simulink model "ControlSystem"  (R2024a)
settings: Solver=FixedStepAuto  StartTime=0.0  StopTime=data.Timestamp(end)  FixedStep=1/60  RelTol=1e-3
values from neighbouring files (symbols this model uses):
  a_denum = exp(-dt/tau_act)    [SimParam.m]
  a_num = 1 - a_denum    [SimParam.m]
  dt = 1/60    (= 0.0166666666667)    [SimParam.m]
  dx = g.dx    [SimParam.m]
  dy = g.dy    [SimParam.m]
  g_a = p.g    [SimParam.m]
  gx = g.gx    [SimParam.m]
  gy = g.gy    [SimParam.m]
  k_heave = 0.05    [SimParam.m]
  k_surge = 0.15    [SimParam.m]
  k_sway = 0.05    [SimParam.m]
  L_i0 = 0.1    [SimParam.m]
  L_max = 0.1    [SimParam.m]
  L_min = -0.1    [SimParam.m]
  max_deg_Surge = 10    [SimParam.m]
  max_deg_Sway = 5    [SimParam.m]
  thickness = g.t    [SimParam.m]
undefined symbols (not defined in the file or in its folder): DiscIntNeverNeededParam
settings Model: Creator=gusta  LastModifiedBy=gusta

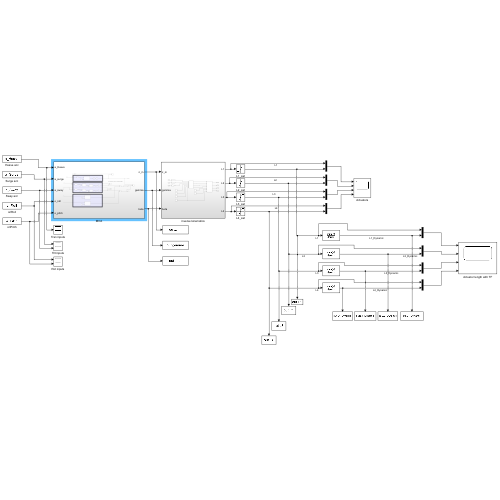
[thumbnail: Simulink's stored preview of the top-level diagram]
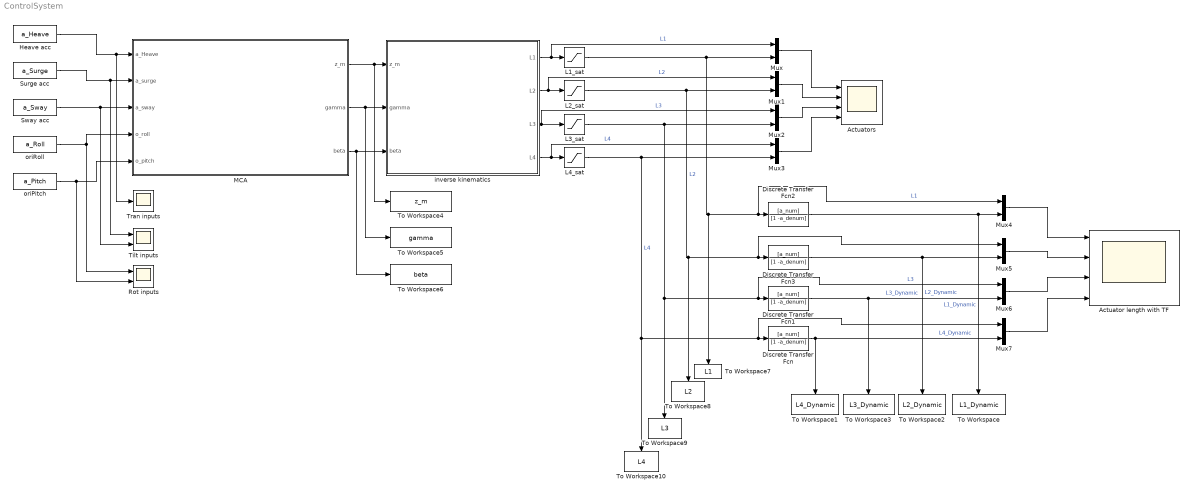
== system ControlSystem ==
  Actuator length with TF : Scope  NumInputPorts=4
  Actuators : Scope  NumInputPorts=4
  Discrete Transfer Fcn{,1..3} (4 alike) : DiscreteTransferFcn  Numerator=[a_num]  Denominator=[1 -a_denum]
  Heave acc : FromWorkspace  VariableName=a_Heave
  L1_sat : Saturate  UpperLimit=L_max  LowerLimit=L_min  ZeroCross=off
  L2_sat : Saturate  UpperLimit=L_max  LowerLimit=L_min  ZeroCross=off
  L3_sat : Saturate  UpperLimit=L_max  LowerLimit=L_min  ZeroCross=off
  L4_sat : Saturate  UpperLimit=L_max  LowerLimit=L_min  ZeroCross=off
  MCA : Subsystem
  Mux{,1..7} (8 alike) : Mux  Inputs=2
  Rot inputs : Scope  NumInputPorts=2
  Surge acc : FromWorkspace  VariableName=a_Surge
  Sway acc : FromWorkspace  VariableName=a_Sway
  Tilt inputs : Scope  NumInputPorts=2
  To Workspace : ToWorkspace  VariableName=L1_Dynamic  SaveFormat=Timeseries  SampleTime=-1
  To Workspace1 : ToWorkspace  VariableName=L4_Dynamic  SaveFormat=Timeseries  SampleTime=-1
  To Workspace10 : ToWorkspace  VariableName=L4  SaveFormat=Timeseries  SampleTime=-1
  To Workspace2 : ToWorkspace  VariableName=L2_Dynamic  SaveFormat=Timeseries  SampleTime=-1
  To Workspace3 : ToWorkspace  VariableName=L3_Dynamic  SaveFormat=Timeseries  SampleTime=-1
  To Workspace4 : ToWorkspace  VariableName=z_m  SaveFormat=Timeseries  SampleTime=-1
  To Workspace5 : ToWorkspace  VariableName=gamma  SaveFormat=Timeseries  SampleTime=-1
  To Workspace6 : ToWorkspace  VariableName=beta  SaveFormat=Timeseries  SampleTime=-1
  To Workspace7 : ToWorkspace  VariableName=L1  SaveFormat=Timeseries  SampleTime=-1
  To Workspace8 : ToWorkspace  VariableName=L2  SaveFormat=Timeseries  SampleTime=-1
  To Workspace9 : ToWorkspace  VariableName=L3  SaveFormat=Timeseries  SampleTime=-1
  Tran inputs : Scope
  inverse kinematics : Subsystem
  oriPitch : FromWorkspace  VariableName=a_Pitch
  oriRoll : FromWorkspace  VariableName=a_Roll
  wires:
  Heave acc/1 -> Tran inputs/1, MCA/1(a_Heave)
  Surge acc/1 -> Tilt inputs/1, MCA/2(a_surge)
  Sway acc/1 -> Tilt inputs/2, MCA/3(a_sway)
  oriRoll/1 -> Rot inputs/1, MCA/4(o_roll)
  oriPitch/1 -> Rot inputs/2, MCA/5(o_pitch)
  MCA/1(z_m) -> To Workspace4/1, inverse kinematics/1(z_m)
  MCA/2(gamma) -> To Workspace5/1, inverse kinematics/2(gamma)
  MCA/3(beta) -> To Workspace6/1, inverse kinematics/3(beta)
  inverse kinematics/4(L4) -> Mux3/1, L4_sat/1  "L4"
  inverse kinematics/3(L3) -> Mux2/1, L3_sat/1  "L3"
  inverse kinematics/2(L2) -> Mux1/1, L2_sat/1  "L2"
  L1_sat/1 -> Mux/2, Mux4/1, Discrete Transfer Fcn2/1, To Workspace7/1  "L1"
  L2_sat/1 -> Mux1/2, Discrete Transfer Fcn3/1, Mux5/1, To Workspace8/1  "L2"
  L3_sat/1 -> Mux2/2, Discrete Transfer Fcn1/1, Mux6/1, To Workspace9/1  "L3"
  L4_sat/1 -> Mux3/2, Mux7/1, Discrete Transfer Fcn/1, To Workspace10/1  "L4"
  inverse kinematics/1(L1) -> Mux/1, L1_sat/1  "L1"
  Mux/1 -> Actuators/1
  Mux1/1 -> Actuators/2
  Mux2/1 -> Actuators/3
  Mux3/1 -> Actuators/4
  Discrete Transfer Fcn2/1 -> To Workspace/1, Mux4/2  "L1_Dynamic"
  Discrete Transfer Fcn3/1 -> Mux5/2, To Workspace2/1  "L2_Dynamic"
  Discrete Transfer Fcn1/1 -> Mux6/2, To Workspace3/1  "L3_Dynamic"
  Discrete Transfer Fcn/1 -> Mux7/2, To Workspace1/1  "L4_Dynamic"
  Mux4/1 -> Actuator length with TF/1
  Mux5/1 -> Actuator length with TF/2
  Mux6/1 -> Actuator length with TF/3
  Mux7/1 -> Actuator length with TF/4

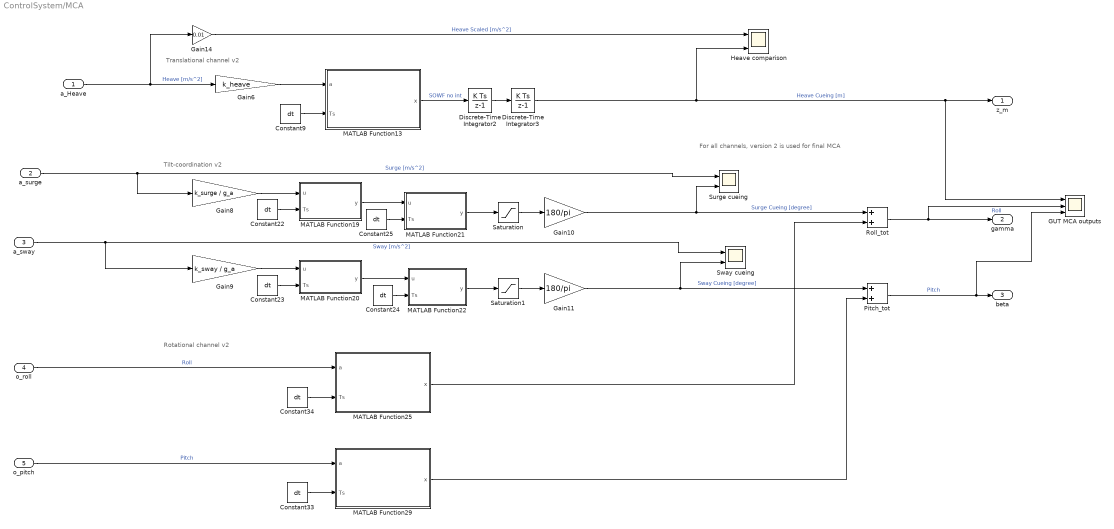
== system ControlSystem/MCA ==
  note: For all channels, version 2 is used for final MCA
  note: Rotational channel v2
  note: Tilt-coordination v2
  note: Translational channel v2
  a_Heave : Inport
  a_surge : Inport  Port=2
  a_sway : Inport  Port=3
  o_roll : Inport  Port=4
  o_pitch : Inport  Port=5
  Constant{9,22..25,33..34} (7 alike) : Constant  Value=dt
  Discrete-Time Integrator2 : DiscreteIntegrator  SampleTime=dt  ICPrevOutput=DiscIntNeverNeededParam  ICPrevScaledInput=DiscIntNeverNeededParam
  Discrete-Time Integrator3 : DiscreteIntegrator  SampleTime=dt  ICPrevOutput=DiscIntNeverNeededParam  ICPrevScaledInput=DiscIntNeverNeededParam
  GUT MCA outputs : Scope  NumInputPorts=3
  Gain10 : Gain  Gain=180/pi
  Gain11 : Gain  Gain=180/pi
  Gain14 : Gain  Gain=0.01
  Gain6 : Gain  Gain=k_heave
  Gain8 : Gain  Gain=k_surge / g_a
  Gain9 : Gain  Gain=k_sway / g_a
  Heave comparison : Scope  NumInputPorts=2
  MATLAB Function13 : MATLAB Function  TreatAsAtomicUnit=on
  MATLAB Function19 : MATLAB Function  TreatAsAtomicUnit=on
  MATLAB Function20 : MATLAB Function  TreatAsAtomicUnit=on
  MATLAB Function21 : MATLAB Function  TreatAsAtomicUnit=on
  MATLAB Function22 : MATLAB Function  TreatAsAtomicUnit=on
  MATLAB Function25 : MATLAB Function  TreatAsAtomicUnit=on
  MATLAB Function29 : MATLAB Function  TreatAsAtomicUnit=on
  Pitch_tot : Sum
  Roll_tot : Sum
  Saturation : Saturate  UpperLimit=max_deg_Surge*pi/180  LowerLimit=-max_deg_Surge*pi/180
  Saturation1 : Saturate  UpperLimit=max_deg_Sway*pi/180  LowerLimit=-max_deg_Sway*pi/180
  Surge cueing : Scope  NumInputPorts=2
  Sway cueing : Scope  NumInputPorts=2
  z_m : Outport
  gamma : Outport  Port=2
  beta : Outport  Port=3
  wires:
  Roll_tot/1 -> gamma/1, GUT MCA outputs/2  "Roll"
  a_surge/1 -> Gain8/1, Surge cueing/1  "Surge [m/s^2]"
  Pitch_tot/1 -> GUT MCA outputs/3, beta/1  "Pitch"
  o_roll/1 -> MATLAB Function25/1(a)  "Roll"
  a_sway/1 -> Gain9/1, Sway cueing/1  "Sway [m/s^2]"
  Constant9/1 -> MATLAB Function13/2(Ts)
  MATLAB Function13/1(x) -> Discrete-Time Integrator2/1  "SOWF no int"
  Gain6/1 -> MATLAB Function13/1(a)
  Constant22/1 -> MATLAB Function19/2(Ts)
  Constant23/1 -> MATLAB Function20/2(Ts)
  Constant25/1 -> MATLAB Function21/2(Ts)
  MATLAB Function20/1(y) -> MATLAB Function22/1(u)
  MATLAB Function19/1(y) -> MATLAB Function21/1(u)
  Gain9/1 -> MATLAB Function20/1(u)
  Gain8/1 -> MATLAB Function19/1(u)
  Constant24/1 -> MATLAB Function22/2(Ts)
  MATLAB Function21/1(y) -> Saturation/1
  MATLAB Function22/1(y) -> Saturation1/1
  Gain10/1 -> Roll_tot/1, Surge cueing/2  "Surge Cueing [degree]"
  Gain11/1 -> Pitch_tot/1, Sway cueing/2  "Sway Cueing [degree]"
  Saturation/1 -> Gain10/1
  Saturation1/1 -> Gain11/1
  o_pitch/1 -> MATLAB Function29/1(a)  "Pitch"
  a_Heave/1 -> Gain14/1, Gain6/1  "Heave [m/s^2]"
  MATLAB Function25/1(x) -> Roll_tot/2
  MATLAB Function29/1(x) -> Pitch_tot/2
  Discrete-Time Integrator2/1 -> Discrete-Time Integrator3/1
  Discrete-Time Integrator3/1 -> Heave comparison/2, z_m/1, GUT MCA outputs/1  "Heave Cueing [m]"
  Constant33/1 -> MATLAB Function29/2(Ts)
  Constant34/1 -> MATLAB Function25/2(Ts)
  Gain14/1 -> Heave comparison/1  "Heave Scaled [m/s^2]"

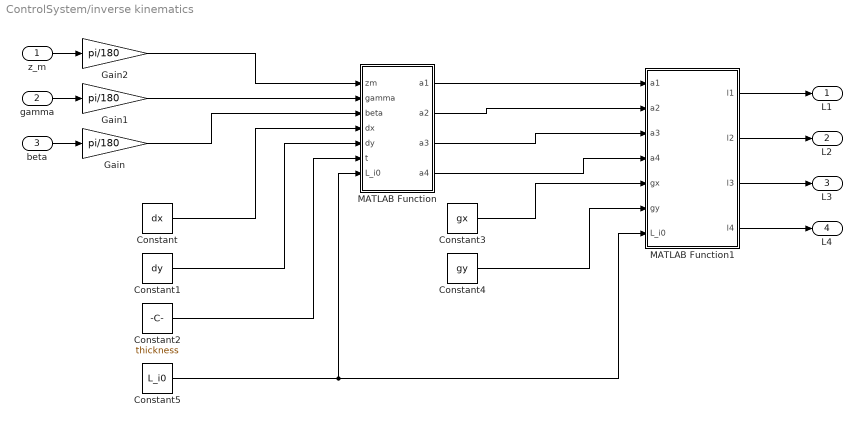
== system ControlSystem/inverse kinematics ==
  z_m : Inport
  gamma : Inport  Port=2
  beta : Inport  Port=3
  Constant : Constant  Value=dx
  Constant1 : Constant  Value=dy
  Constant2 : Constant  Value=thickness
  Constant3 : Constant  Value=gx
  Constant4 : Constant  Value=gy
  Constant5 : Constant  Value=L_i0
  Gain : Gain  Gain=pi/180
  Gain1 : Gain  Gain=pi/180
  Gain2 : Gain  Gain=pi/180
  MATLAB Function : MATLAB Function  TreatAsAtomicUnit=on
  MATLAB Function1 : MATLAB Function  TreatAsAtomicUnit=on
  L1 : Outport
  L2 : Outport  Port=2
  L3 : Outport  Port=3
  L4 : Outport  Port=4
  wires:
  Constant/1 -> MATLAB Function/4(dx)
  Constant1/1 -> MATLAB Function/5(dy)
  Constant2/1 -> MATLAB Function/6(t)
  z_m/1 -> Gain2/1
  gamma/1 -> Gain1/1
  beta/1 -> Gain/1
  MATLAB Function/1(a1) -> MATLAB Function1/1(a1)
  MATLAB Function/2(a2) -> MATLAB Function1/2(a2)
  MATLAB Function/3(a3) -> MATLAB Function1/3(a3)
  MATLAB Function/4(a4) -> MATLAB Function1/4(a4)
  Constant3/1 -> MATLAB Function1/5(gx)
  Constant4/1 -> MATLAB Function1/6(gy)
  MATLAB Function1/1(l1) -> L1/1
  MATLAB Function1/2(l2) -> L2/1
  MATLAB Function1/3(l3) -> L3/1
  MATLAB Function1/4(l4) -> L4/1
  Gain2/1 -> MATLAB Function/1(zm)
  Gain1/1 -> MATLAB Function/2(gamma)
  Gain/1 -> MATLAB Function/3(beta)
  Constant5/1 -> MATLAB Function1/7(L_i0), MATLAB Function/7(L_i0)

== matlab function ControlSystem/inverse kinematics/MATLAB Function ==
  data: zm input; gamma input; beta input; a1 output; dx input; dy input; a2 output; a3 output; a4 output; t input; L_i0 input
function [a1, a2, a3, a4] = fcn(zm, gamma, beta, dx, dy, t, L_i0)
z_m_abs = zm + L_i0 + t/2;
C_M = [0; 0; z_m_abs];
d1 = [dx; -dy; -t/2];
d2 = [-dx; -dy; -t/2];
d3 = [dx; dy; -t/2];
d4 = [-dx; dy; -t/2];

R = [cos(beta)     sin(beta)*sin(gamma)   sin(beta)*cos(gamma);
         0          cos(gamma)          -sin(gamma);
         -sin(beta)    cos(beta)*sin(gamma)   cos(beta)*cos(gamma)];

a1 = C_M + R*d1;
a2 = C_M + R*d2;
a3 = C_M + R*d3;
a4 = C_M + R*d4;

== matlab function ControlSystem/inverse kinematics/MATLAB Function1 ==
  data: a1 input; l1 output; a2 input; a3 input; a4 input; l2 output; l3 output; l4 output; gx input; gy input; L_i0 input
function [l1, l2, l3, l4] = fcn(a1, a2, a3, a4, gx, gy, L_i0)

G1 = [ gx; -gy; 0];
G2 = [-gx; -gy; 0];
G3 = [ gx;  gy; 0];
G4 = [-gx;  gy; 0];

l1 = norm(a1 - G1) - L_i0;
l2 = norm(a2 - G2) - L_i0;
l3 = norm(a3 - G3) - L_i0;
l4 = norm(a4 - G4) - L_i0;

== matlab function ControlSystem/MCA/MATLAB Function13 ==
  data: a input; x output; Ts input
function x = second_order_hpf(a, Ts)
%#codegen
% Second-order high-pass filter from acceleration to position
% Inputs:
%   a  - acceleration input (scalar)
%   Ts - sample time [s]

% Tuning parameters
amax = 20;       % max expected acceleration [m/s^2]
xmax = 0.02;     % max allowed excursion [m]
zeta = 0.7;      % damping ratio

% Compute filter constants
wn = sqrt(0.01*amax / xmax);         % natural frequency [rad/s]

k1 = 2 * zeta * wn;
k2 = wn^2;

persistent x1 x2 a1 a2
if isempty(x1)
    x1 = 0; % x[k-1]
    x2 = 0; % x[k-2]
    a1 = 0; % a[k-1]
    a2 = 0; % a[k-2]
end

% Discrete-time filter coefficients (Tustin approximation)
T = Ts;
b0 = 4 / T^2;
b1 = -8 / T^2;
b2 = 4 / T^2;

a0 = b0 + k1 * 2 / T + k2;
a1d = -2 * b0 + 2 * k2;
a2d = b0 - k1 * 2 / T + k2;

% Difference equation:
x = (b0*a + b1*a1 + b2*a2 - a1d*x1 - a2d*x2) / a0;

% Update history
a2 = a1;
a1 = a;
x2 = x1;
x1 = x;
end

== matlab function ControlSystem/MCA/MATLAB Function19 ==
  data: u input; y output; Ts input
function y = lowpass2(u, Ts)
persistent y1 y2
fc = 0.2;
if isempty(y1)
    y1 = 0; % Initial condition
    y2 = 0;
end

tau = 1 / (2 * pi * fc);
alpha = Ts / (tau + Ts);

y1 = y1 + alpha * (u - y1);

y2 = y2 + alpha * (y1 - y2);

y = y2;
end

== matlab function ControlSystem/MCA/MATLAB Function20 ==
  data: u input; y output; Ts input
function y = lowpass2(u, Ts)
persistent y1 y2
fc = 0.2;
if isempty(y1)
    y1 = 0; % Initial condition
    y2 = 0;
end

tau = 1 / (2 * pi * fc);
alpha = Ts / (tau + Ts);

y1 = y1 + alpha * (u - y1);

y2 = y2 + alpha * (y1 - y2);

y = y2;
end

== matlab function ControlSystem/MCA/MATLAB Function21 ==
  data: u input; y output; Ts input
function y = RateLimiter(u, Ts)
persistent y_prev
S_up = 8 * pi/180;
S_down = 8 * pi/180;

if isempty(y_prev)
    y_prev = 0;
end

y_max = y_prev + S_up * Ts;
y_min = y_prev - S_down * Ts;

y = min(max(u, y_min), y_max);
y_prev = y;
end

== matlab function ControlSystem/MCA/MATLAB Function22 ==
  data: u input; y output; Ts input
function y = RateLimiter(u, Ts)
persistent y_prev
S_up = 8 * pi/180;
S_down = 8 * pi/180;

if isempty(y_prev)
    y_prev = 0;
end

y_max = y_prev + S_up * Ts;
y_min = y_prev - S_down * Ts;

y = min(max(u, y_min), y_max);
y_prev = y;
end

== matlab function ControlSystem/MCA/MATLAB Function25 ==
  data: a input; x output; Ts input
function x = second_order_hpf(a, Ts)
%#codegen
% Second-order high-pass filter from acceleration to position
% Inputs:
%   a  - acceleration input (scalar)
%   Ts - sample time [s]

% Tuning parameters
amax = 3.16;       % max expected acceleration [m/s^2]
xmax = 0.02;     % max allowed excursion [m]
zeta = 0.7;      % damping ratio

% Compute filter constants
%wn = sqrt(0.01*amax / xmax);         % natural frequency [rad/s]
wn = 1.257;         % Natural frequency wn = 2*pi*fc

k1 = 2 * zeta * wn;
k2 = wn^2;

persistent x1 x2 a1 a2
if isempty(x1)
    x1 = 0; % x[k-1]
    x2 = 0; % x[k-2]
    a1 = 0; % a[k-1]
    a2 = 0; % a[k-2]
end

% Discrete-time filter coefficients (Tustin approximation)
T = Ts;
b0 = 4 / T^2;
b1 = -8 / T^2;
b2 = 4 / T^2;

a0 = b0 + k1 * 2 / T + k2;
a1d = -2 * b0 + 2 * k2;
a2d = b0 - k1 * 2 / T + k2;

% Difference equation:
x = (b0*a + b1*a1 + b2*a2 - a1d*x1 - a2d*x2) / a0;

% Update history
a2 = a1;
a1 = a;
x2 = x1;
x1 = x;
end

== matlab function ControlSystem/MCA/MATLAB Function29 ==
  data: a input; x output; Ts input
function x = second_order_hpf(a, Ts)
%#codegen
% Second-order high-pass filter from acceleration to position
% Inputs:
%   a  - acceleration input (scalar)
%   Ts - sample time [s]

% Tuning parameters
amax = 20;       % max expected acceleration [m/s^2]
xmax = 0.02;     % max allowed excursion [m]
zeta = 0.7;      % damping ratio

% Compute filter constants
%wn = sqrt(0.01*amax / xmax);         % natural frequency [rad/s]
wn = 1.257;         % Natural frequency wn = 2*pi*fc

k1 = 2 * zeta * wn;
k2 = wn^2;

persistent x1 x2 a1 a2
if isempty(x1)
    x1 = 0; % x[k-1]
    x2 = 0; % x[k-2]
    a1 = 0; % a[k-1]
    a2 = 0; % a[k-2]
end

% Discrete-time filter coefficients (Tustin approximation)
T = Ts;
b0 = 4 / T^2;
b1 = -8 / T^2;
b2 = 4 / T^2;

a0 = b0 + k1 * 2 / T + k2;
a1d = -2 * b0 + 2 * k2;
a2d = b0 - k1 * 2 / T + k2;

% Difference equation:
x = (b0*a + b1*a1 + b2*a2 - a1d*x1 - a2d*x2) / a0;

% Update history
a2 = a1;
a1 = a;
x2 = x1;
x1 = x;
end
